simulink model "spektr_scope1"  (Simulink 7.8)
settings: Solver=ode45  StartTime=0.0  StopTime=10.0  RelTol=1e-3
undefined symbols (not defined in the file or in its folder): Buffer, D, dfilt, dspbuff3, get, navg, UseBuffer
libraries: dspsnks4 x3, dspspect3 x2, dspmisc x2, dsparch4 x1, dspsigattribs x1, dspsigops x1
settings Model: Creator=svenhoffmann  LastModifiedBy=josef  ExtModeAutoUpdateStatusClock=off
settings OptimizationCC: InitFltsAndDblsToZero=on
settings DebuggingCC: SaveWithParameterizedLinksMsg=none  SignalResolutionControl=TryResolveAllWithWarning  MultiTaskDSMMsg=warning  MultiTaskCondExecSysMsg=none  FcnCallInpInsideContextMsg=Use local settings  StrictBusMsg=None
settings RTWCC: IncludeERTFirstTime=on
settings GRTTargetCC: TargetFcnLib=ansi_tfl_tmw.mat

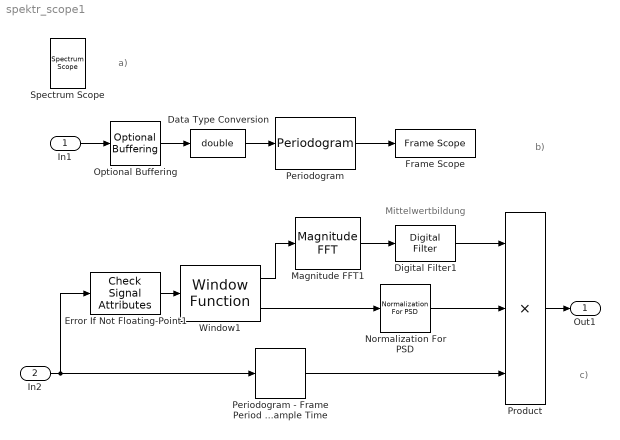
== system spektr_scope1 ==
  note: a)
  note: b)
  note: c)
  note: Mittelwertbildung
  In1 : Inport
  In2 : Inport  Port=2
  Data Type Conversion : DataTypeConversion  OutDataTypeStr=double  SaturateOnIntegerOverflow=on  RndMeth=Zero
  Digital Filter1 : dsparch4/Digital Filter  TypePopup=FIR (all zeros)  IIRFiltStruct=Direct form II transposed  AllPoleFiltStruct=Direct form  FIRFiltStruct=Direct form  CoeffSource=Specify via dialog  NumCoeffs=ones(navg,1)/navg  DenCoeffs=[1 0.1]  BiQuadCoeffs=[1 0.3 0.4 1 0.1 0.2]  LatticeCoeffs=[0.2 0.4]  denIgnore=on  FiltPerSampPopup=One filter per frame  IC=0  ICnum=0  ICden=0  roundingMode=Floor  overflowMode=off  ScaleValues=1  scaleValueFracLength=14  stageInFracLength=15  stageOutFracLength=15  FilterSource=Specify via dialog  dfiltObjectName=dfilt.dffir([1 2 1])
  Error If Not Floating-Point1 : dspsigattribs/Check Signal Attributes  SigAttribCheckMethod=Does not match attributes exactly  Complexity=Ignore  Frame=Ignore  DimsCheckMethod=Ignore  Dimensions=1-D  DatatypeCheckMethod=Is...  DatatypeGeneral=Floating-point  DtypeFloatSpecific=Any floating-point  DtypeFixedSpecific=Any fixed-point  DtypeIntSpecific=Any integer  SampleMode=Ignore
  Frame Scope : dspsnks4/Spectrum Scope/Frame Scope
  Magnitude FFT1 : dspspect3/Magnitude FFT  mag_or_magsq=Magnitude squared  FFTImplementation=Auto  fftLenInherit=off  fftsize=fftsize
  Normalization For PSD : dspmisc/Normalization For PSD
  Optional Buffering : dspsnks4/Spectrum Scope/Optional Buffering  oname=Buffer  osrc=dspbuff3/Buffer  oargs={'N','BufferSize','V','Overlap','ic','0'}  replace=strcmp(UseBuffer,'off')
  Periodogram : dspspect3/Periodogram  measurement=Power spectral density  wintype=Hann  Rs=RsSpecScope  beta=betaSpecScope  winsamp=Periodic  FFTImplementation=Auto  inheritFFT=on  fftsize=FFTlength  navg=numAvg  inheritTs=on  Ts=1
  Periodogram - Frame Period To Sample Time : dspmisc/Periodogram - Frame Period To Sample Time
  Product : Product  Inputs=***  SaturateOnIntegerOverflow=on  InputSameDT=on  OutDataTypeStr=Inherit: Same as first input
  Spectrum Scope : dspsnks4/Spectrum Scope  ScopeProperties=on  Domain=Frequency  HorizSpan=1  UseBuffer=off  BufferSize=128  Overlap=64  TreatMby1Signals=One channel  inpFftLenInherit=off  FFTlength=128  numAvg=2  DisplayProperties=off  AxisGrid=on  Memory=off  FrameNumber=on  AxisLegend=off  AxisZoom=off  OpenScopeAtSimStart=on  OpenScopeImmediately=off  FigPos=get(0,'defaultfigureposition')  AxisProperties=off  XUnits=Hertz  XRange=[0...Fs/2]  XDisplay=0  InheritXIncr=on  XIncr=1.0  XLabel=Samples  XLimit=Auto  YUnits=dB  XMax=1  XMin=0  YLabel=Magnitude-squared, dB  LineProperties=off  wintypeSpecScope=Hann  RsSpecScope=50  betaSpecScope=5  winsampSpecScope=Periodic  XAxisParamsVer=6.8  isFrameUpgraded=on
      settings: YMin=-10  YMax=10
  Window1 : dspsigops/Window Function  winmode=Generate and apply window  wintype=Hann  sampmode=Continuous  samptime=1  N=64  Rs=Rs  beta=beta  winsamp=Periodic  UserWindow=hamming  OptParams=off  UserParams={1.0}  RowConvenienceOn=off  dataType=double  isSigned=on  wordLen=16  udDataType=sfix(16)  fracBitsMode=Best precision  numFracBits=15  roundingMode=Floor  overflowMode=off  numSidelobes=4  sidelobeLevel=-30
      settings: additionalParams=on
  Out1 : Outport  InitialOutput=0
  wires:
  Periodogram/1 -> Frame Scope/1
  In1/1 -> Optional Buffering/1
  Optional Buffering/1 -> Data Type Conversion/1
  Data Type Conversion/1 -> Periodogram/1
  Periodogram - Frame Period To Sample Time/1 -> Product/3
  Error If Not Floating-Point1/1 -> Window1/1
  Window1/2 -> Normalization For PSD/1
  Normalization For PSD/1 -> Product/2
  Digital Filter1/1 -> Product/1
  Product/1 -> Out1/1
  Window1/1 -> Magnitude FFT1/1
  Magnitude FFT1/1 -> Digital Filter1/1
  In2/1 -> Error If Not Floating-Point1/1, Periodogram - Frame Period To Sample Time/1
